simulink model "CSlab2"  (R2017a)
settings: Solver=ode45  StartTime=0.0  StopTime=10.0  RelTol=1e-3  EnableMultiTasking=on
PreLoadFcn:
  | % Motor Parameters
  | 
  | J=0.01;     %kg*m^2
  | b=0.1;      %N*m/(rad/s)
  | K=0.01;     %V/(rad/s)
  | R=1;        %Ohm
  | L=0.5;      %H
libraries: simulink x1
settings Model: Creator=deastman  LastModifiedBy=HP
settings DataIOCC: LimitDataPoints=on  SaveFormat=Array  SignalLoggingSaveFormat=ModelDataLogs
settings OptimizationCC: ExpressionDepthLimit=2147483647  InitFltsAndDblsToZero=on  LifeSpan=inf
settings DebuggingCC: UnderspecifiedInitializationDetection=Classic  MergeDetectMultiDrivingBlocksExec=none  SolverPrmCheckMsg=warning  FcnCallInpInsideContextMsg=warning  StateNameClashWarn=warning  SFUnexpectedBacktrackingDiag=warning  SFNoUnconditionalDefaultTransitionDiag=warning  SFExecutionAtInitializationDiag=none
settings HardwareCC: ProdBitPerPointer=32  ProdBitPerSizeT=32  ProdBitPerPtrDiffT=32  ProdLargestAtomicFloat=None  ProdIntDivRoundTo=Undefined  ProdEndianess=Unspecified  ProdWordSize=32  ProdHWDeviceType=32-bit Generic
settings ModelReferenceCC: PropagateSignalLabelsOutOfModel=off
settings GRTTargetCC: TargetLangStandard=C89/C90 (ANSI)  GeneratePreprocessorConditionals=Disable all  CombineOutputUpdateFcns=off  GRTInterface=on
settings ConfigComp: CovMetricSettings=dw  CovHtmlReporting=on  CovSaveCumulativeToWorkspaceVar=on  CovSaveSingleToWorkspaceVar=on  CovExternalEMLEnable=off  CovSFcnEnable=off

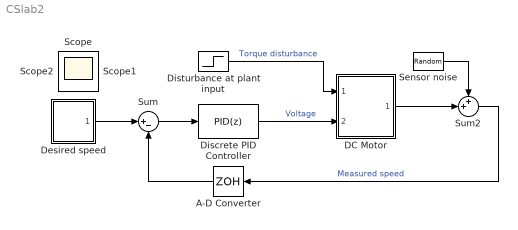
== system CSlab2 ==
  " Disturbance at plant input" : Step  Time=5  After=0.2  SampleTime=0
  A-D Converter : ZeroOrderHold  SampleTime=0.02
  DC Motor : Subsystem  mask(DC Motor){b=b, J=J, K=K, R=R, L=L}
      mask prompts: b "Damping:"; J "Inertia:"; K "Back EMF:"; R "Resistance:"; L "Inductance:"
      mask help: An ideal model of a DC Motor
      mask Help: This is <b>more elaborate<b> help.
      mask Display: image(imread('dcmotor.jpg'))
  Desired speed : Subsystem
  Discrete PID Controller : simulink/Continuous/PID Controller  Controller=PID  TimeDomain=Discrete-time  SampleTime=0.02  IntegratorMethod=Forward Euler  FilterMethod=Forward Euler  Form=Parallel  UseFilter=on  ControllerParametersSource=internal  P=17.6352849318875  I=46.1002596426595  D=0.961635498325191  N=79.036730484224  InitialConditionSource=internal  InitialConditionForIntegrator=0  InitialConditionForFilter=0  ExternalReset=none  LimitOutput=off  UpperSaturationLimit=10  LowerSaturationLimit=-10  LinearizeAsGain=on  AntiWindupMode=back-calculation  Kb=1  TrackingMode=off  Kt=1  PParamMin=[]  PParamMax=[]  IParamMin=[]  IParamMax=[]  DParamMin=[]  DParamMax=[]  NParamMin=[]  NParamMax=[]  KbParamMin=[]  KbParamMax=[]  KtParamMin=[]  KtParamMax=[]  POutMin=[]  POutMax=[]  IOutMin=[]  IOutMax=[]  DOutMin=[]  DOutMax=[]  NOutMin=[]  NOutMax=[]  KbOutMin=[]  KbOutMax=[]  KtOutMin=[]  KtOutMax=[]  IntegratorOutMin=[]  IntegratorOutMax=[]  FilterOutMin=[]  FilterOutMax=[]  SumOutMin=[]  SumOutMax=[]  SumI1OutMin=[]  SumI1OutMax=[]  SumI2OutMin=[]  SumI2OutMax=[]  SumI3OutMin=[]  SumI3OutMax=[]  SumDOutMin=[]  SumDOutMax=[]  SaturationOutMin=[]  SaturationOutMax=[]  IntegratorContinuousStateAttributes=''  IntegratorStateMustResolveToSignalObject=off  IntegratorRTWStateStorageClass=Auto  FilterContinuousStateAttributes=''  FilterStateMustResolveToSignalObject=off  FilterRTWStateStorageClass=Auto  DifferentiatorICPrevScaledInput=0  DifferentiatorOutMin=[]  DifferentiatorOutMax=[]  InitialConditionSetting=State (most efficient)
  Sensor noise : RandomNumber  Variance=0.05  SampleTime=0
  Sum : Sum  Inputs=|+-
  Sum2 : Sum  Inputs=++|
  Scope : Scope
  Scope1 : Scope
  Scope2 : Scope
  wires:
  " Disturbance at plant input"/1 -> DC Motor/1(Torque)  "Torque disturbance"
  Sum/1 -> Discrete PID Controller/1
  Discrete PID Controller/1 -> DC Motor/2(Voltage)  "Voltage"
  Desired speed/1(Speed) -> Sum/1
  DC Motor/1(Speed) -> Sum2/2
  Sum2/1 -> A-D Converter/1  "Measured speed"
  Sensor noise/1 -> Sum2/1
  A-D Converter/1 -> Sum/2

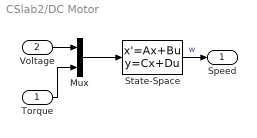
== system CSlab2/DC Motor ==
  Torque : Inport
  Voltage : Inport  Port=2
  Mux : Mux  Inputs=2
  State-Space : StateSpace  A=[-b/J K/J; -K/L -R/L]  B=[0 -1/J; 1/L 0]  C=[1 0]  D=[0 0]  X0=0
  Speed : Outport
  wires:
  Mux/1 -> State-Space/1
  Voltage/1 -> Mux/1
  State-Space/1 -> Speed/1  "w"
  Torque/1 -> Mux/2

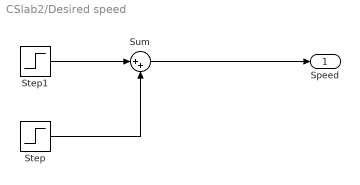
== system CSlab2/Desired speed ==
  Step : Step  Time=7  After=-4  SampleTime=0.02
  Step1 : Step  After=2  SampleTime=0.02
  Sum : Sum  Inputs=|++
  Speed : Outport
  wires:
  Step/1 -> Sum/2
  Step1/1 -> Sum/1
  Sum/1 -> Speed/1
